simulink subsystem "controleLEDbyTactSw"  (R2020b)
settings: Solver=VariableStepAuto  StartTime=0.0  StopTime=10.0  RelTol=1e-3
settings Model: Creator=kitaw  LastModifiedBy=kitaw

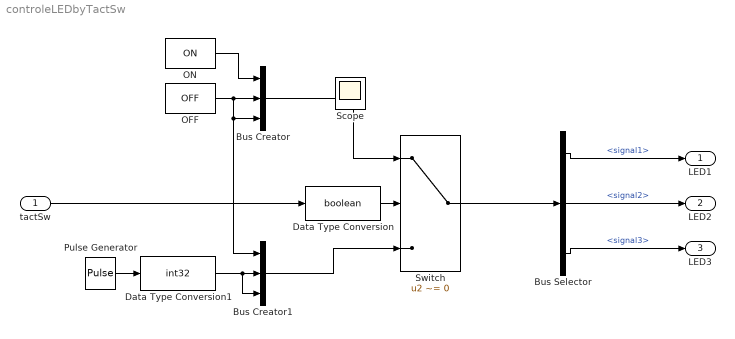
== system controleLEDbyTactSw ==
  tactSw : Inport
  Bus Creator : BusCreator  Inputs=3
  Bus Creator1 : BusCreator  Inputs=3
  Bus Selector : BusSelector  OutputSignals=signal1,signal2,signal3
  Data Type Conversion : DataTypeConversion  OutDataTypeStr=boolean
  Data Type Conversion1 : DataTypeConversion  OutDataTypeStr=int32
  OFF : Constant  Value=OFF  SampleTime=-1
  ON : Constant  Value=ON  SampleTime=-1
  Pulse Generator : DiscretePulseGenerator  PulseType=Time based  Period=6  PulseWidth=50
  Switch : Switch  Criteria=u2 ~= 0
  LED1 : Outport
  LED2 : Outport  Port=2
  LED3 : Outport  Port=3
  Scope : Scope
  wires:
  Data Type Conversion/1 -> Switch/2
  tactSw/1 -> Data Type Conversion/1
  ON/1 -> Bus Creator/1
  OFF/1 -> Bus Creator/2, Bus Creator/3, Bus Creator1/1
  Bus Creator/1 -> Switch/1
  Pulse Generator/1 -> Data Type Conversion1/1
  Data Type Conversion1/1 -> Bus Creator1/2, Bus Creator1/3
  Bus Creator1/1 -> Switch/3
  Switch/1 -> Bus Selector/1
  Bus Selector/1 -> LED1/1  "<signal1>"
  Bus Selector/2 -> LED2/1  "<signal2>"
  Bus Selector/3 -> LED3/1  "<signal3>"
